simulink model "meam_simulink"  (R2020a)
settings: Solver=FixedStepAuto  StartTime=0.0  StopTime=10.0  FixedStep=0.0001  RelTol=1e-3
undefined symbols (not defined in the file): cnc_comp, ctc_switch, ctrl_at_end, ctrl_space, delta, ea_set_1, ea_set_2, ee_att_1, ee_att_2, f_des, force_ffwd, fp_1, fp_2, frc_comp, grv_comp, ip_1, ip_2, K, Kc, Kd, Kdf, Ki, Kif, Km, Kp, Kpf, orn_at_norm, prdc_frc, q_posIni, q_posIni_1, robot_model_1, robot_model_2, rpt_num_1, rpt_num_2, Sf_diag, spr_comp, switch_val, Sx_diag, tf_1, tf_2, trj_at_end, trj_profile_1, trj_profile_2, trj_space_1, trj_space_2, trj_type_1, trj_type_2
libraries: simulink x2, vrlib x1
(part 2 of 4)

== system meam_simulink/Subsystem/End-to-Base ==
  y : Inport  PortDimensions=6
  des : Inport  Port=2  PortDimensions=30
  fbk : Inport  Port=3  PortDimensions=30
  Constant2 : Constant  Value=ctrl_at_end
  Demux : Demux  Outputs=[12;18]
  Demux1 : Demux  Outputs=[12;18]
  Demux2 : Demux  Outputs=[12;6]
  Switch : Switch  Criteria=u2 > Threshold
  Terminator : Terminator
  Terminator1 : Terminator
  computed torque switch : Constant  Value=ctc_switch
  spatialTrnsE2B : MATLAB Function  TreatAsAtomicUnit=on
  u : Outport  PortDimensions=6
  wires:
  y/1 -> spatialTrnsE2B/5(u), Switch/3
  spatialTrnsE2B/1(y) -> Switch/1
  Constant2/1 -> Switch/2
  des/1 -> Demux/1
  Demux/1 -> spatialTrnsE2B/1(q)
  Demux/2 -> spatialTrnsE2B/2(x)
  Switch/1 -> u/1
  computed torque switch/1 -> spatialTrnsE2B/4(ctc_switch)
  fbk/1 -> Demux1/1
  Demux1/2 -> Demux2/1
  Demux2/2 -> spatialTrnsE2B/3(v)
  Demux1/1 -> Terminator/1
  Demux2/1 -> Terminator1/1

== system meam_simulink/Subsystem/End-to-Base Wrench ==
  y : Inport  PortDimensions=6
  des : Inport  Port=2  PortDimensions=30
  Constant2 : Constant  Value=ctrl_at_end
  Demux : Demux  Outputs=[12;18]
  Switch : Switch  Criteria=u2 > Threshold
  Terminator : Terminator
  spatialTrnsE2B : MATLAB Function  TreatAsAtomicUnit=on
  u : Outport  PortDimensions=6
  wires:
  y/1 -> Switch/3, spatialTrnsE2B/2(f_desE)
  spatialTrnsE2B/1(f_des) -> Switch/1
  Constant2/1 -> Switch/2
  des/1 -> Demux/1
  Demux/2 -> spatialTrnsE2B/1(x)
  Switch/1 -> u/1
  Demux/1 -> Terminator/1

== system meam_simulink/Subsystem/Error ==
  des : Inport  PortDimensions=30
  fbk : Inport  Port=2  PortDimensions=30
  Demux : Demux  Outputs=[12;18]
  Demux1 : Demux  Outputs=[12;18]
  MATLAB Function : MATLAB Function  TreatAsAtomicUnit=on
  Sum : Sum  Inputs=|+-
  Switch : Switch  Criteria=u2 > Threshold
  control_space : Constant  Value=ctrl_space
  e : Outport
  wires:
  fbk/1 -> Demux1/1
  des/1 -> Demux/1
  control_space/1 -> Switch/2
  MATLAB Function/1(y) -> Switch/1
  Demux/1 -> Sum/1
  Demux1/1 -> Sum/2
  Sum/1 -> Switch/3
  Demux/2 -> MATLAB Function/1(des)
  Demux1/2 -> MATLAB Function/2(fbk)
  Switch/1 -> e/1

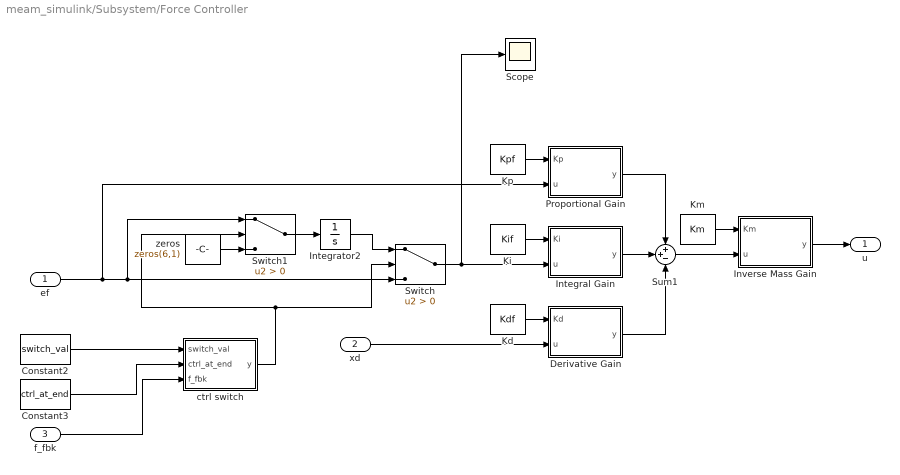
== system meam_simulink/Subsystem/Force Controller ==
  ef : Inport
  xd : Inport  Port=2
  f_fbk : Inport  Port=3
  Constant2 : Constant  Value=switch_val
  Constant3 : Constant  Value=ctrl_at_end
  Derivative Gain : MATLAB Function  TreatAsAtomicUnit=on
  Integral Gain : MATLAB Function  TreatAsAtomicUnit=on
  Integrator2 : Integrator
  Inverse Mass Gain : MATLAB Function  TreatAsAtomicUnit=on
  Kd : Constant  Value=Kdf
  Ki : Constant  Value=Kif
  Km : Constant  Value=Km
  Kp : Constant  Value=Kpf
  Proportional Gain : MATLAB Function  TreatAsAtomicUnit=on
  Scope : Scope
  Sum1 : Sum  Inputs=++-
  Switch : Switch  Criteria=u2 > Threshold
  Switch1 : Switch  Criteria=u2 > Threshold
  ctrl switch : MATLAB Function  TreatAsAtomicUnit=on
  zeros : Constant  Value=zeros(6,1)
  u : Outport
  wires:
  Proportional Gain/1(y) -> Sum1/1
  Integral Gain/1(y) -> Sum1/2
  ef/1 -> Switch/3, Switch1/1, Proportional Gain/2(u)
  Kp/1 -> Proportional Gain/1(Kp)
  Ki/1 -> Integral Gain/1(Ki)
  Kd/1 -> Derivative Gain/1(Kd)
  Derivative Gain/1(y) -> Sum1/3
  xd/1 -> Derivative Gain/2(u)
  Inverse Mass Gain/1(y) -> u/1
  Sum1/1 -> Inverse Mass Gain/2(u)
  Km/1 -> Inverse Mass Gain/1(Km)
  Constant3/1 -> ctrl switch/2(ctrl_at_end)
  Constant2/1 -> ctrl switch/1(switch_val)
  f_fbk/1 -> ctrl switch/3(f_fbk)
  Switch1/1 -> Integrator2/1
  Integrator2/1 -> Switch/1
  zeros/1 -> Switch1/3
  ctrl switch/1(y) -> Switch/2, Switch1/2
  Switch/1 -> Scope/1, Integral Gain/2(u)

== system meam_simulink/Subsystem/Kin Trns ==
  u : Inport
  q_fbk : Inport  Port=2
  Demux : Demux  Outputs=[6;6]
  Demux1 : Demux  Outputs=[12;18]
  MATLAB Function : MATLAB Function  TreatAsAtomicUnit=on
  Switch : Switch  Criteria=u2 > Threshold
  Terminator1 : Terminator
  computed torque switch : Constant  Value=ctc_switch
  control space : Constant  Value=ctrl_space
  end-effector attach : Constant  Value=ee_att_1
  robot_model : Constant  Value=robot_model_1
  y : Outport
  wires:
  u/1 -> Switch/3, MATLAB Function/4(u)
  robot_model/1 -> MATLAB Function/1(robot_model)
  Demux/1 -> MATLAB Function/5(q_pos)
  control space/1 -> Switch/2
  q_fbk/1 -> Demux1/1
  Demux1/1 -> Demux/1
  Demux/2 -> MATLAB Function/6(q_vel)
  Demux1/2 -> Terminator1/1
  Switch/1 -> y/1
  MATLAB Function/1(tau) -> Switch/1
  computed torque switch/1 -> MATLAB Function/3(ctc_switch)
  end-effector attach/1 -> MATLAB Function/2(ee_att)

== system meam_simulink/Subsystem/Motion Controller ==
  e : Inport
  Demux1 : Demux  Outputs=2
  Derivative Gain : MATLAB Function  TreatAsAtomicUnit=on
  Integral Gain : MATLAB Function  TreatAsAtomicUnit=on
  Integrator2 : Integrator
  Inverse Mass Gain : MATLAB Function  TreatAsAtomicUnit=on
  Kd : Constant  Value=Kd
  Ki : Constant  Value=Ki
  Km : Constant  Value=Km
  Kp : Constant  Value=Kp
  Proportional Gain : MATLAB Function  TreatAsAtomicUnit=on
  Scope : Scope
  Sum1 : Sum  Inputs=+++
  u : Outport
  wires:
  Derivative Gain/1(y) -> Sum1/3
  Proportional Gain/1(y) -> Sum1/1
  Integrator2/1 -> Integral Gain/2(u)
  Integral Gain/1(y) -> Sum1/2
  Demux1/2 -> Derivative Gain/2(u)
  e/1 -> Demux1/1
  Demux1/1 -> Scope/1, Proportional Gain/2(u), Integrator2/1
  Kp/1 -> Proportional Gain/1(Kp)
  Ki/1 -> Integral Gain/1(Ki)
  Kd/1 -> Derivative Gain/1(Kd)
  Km/1 -> Inverse Mass Gain/1(Km)
  Inverse Mass Gain/1(y) -> u/1
  Sum1/1 -> Inverse Mass Gain/2(u)

== system meam_simulink/Subsystem/Selective Sum ==
  um : Inport  PortDimensions=6
  uf : Inport  Port=2  PortDimensions=6
  f_fbk : Inport  Port=3  PortDimensions=6
  Constant : Constant  Value=Sx_diag
  Constant1 : Constant  Value=Sf_diag
  Constant2 : Constant  Value=switch_val
  Constant3 : Constant  Value=ctrl_at_end
  MATLAB Function : MATLAB Function  TreatAsAtomicUnit=on
  Out1 : Outport  PortDimensions=6
  wires:
  uf/1 -> MATLAB Function/6(uf)
  um/1 -> MATLAB Function/1(um)
  MATLAB Function/1(y) -> Out1/1
  Constant/1 -> MATLAB Function/2(Sx_diag)
  Constant1/1 -> MATLAB Function/5(Sf_diag)
  Constant2/1 -> MATLAB Function/3(switch_val)
  f_fbk/1 -> MATLAB Function/7(f_fbk)
  Constant3/1 -> MATLAB Function/4(ctrl_at_end)

== system meam_simulink/Subsystem1/Acc Switch ==
  In1 : Inport
  In2 : Inport  Port=2
  Demux : Demux  Outputs=2
  Sum : Sum  Inputs=++|
  Switch : Switch  Criteria=u2 > Threshold
  Switch1 : Switch  Criteria=u2 > Threshold
  computed torque switch : Constant  Value=ctc_switch
  control space : Constant  Value=ctrl_space
  Out1 : Outport
  wires:
  Sum/1 -> Switch/1
  computed torque switch/1 -> Switch/2
  Switch/1 -> Out1/1
  In1/1 -> Switch/3, Sum/1
  Switch1/1 -> Sum/2
  In2/1 -> Demux/1
  Demux/1 -> Switch1/3
  control space/1 -> Switch1/2
  Demux/2 -> Switch1/1

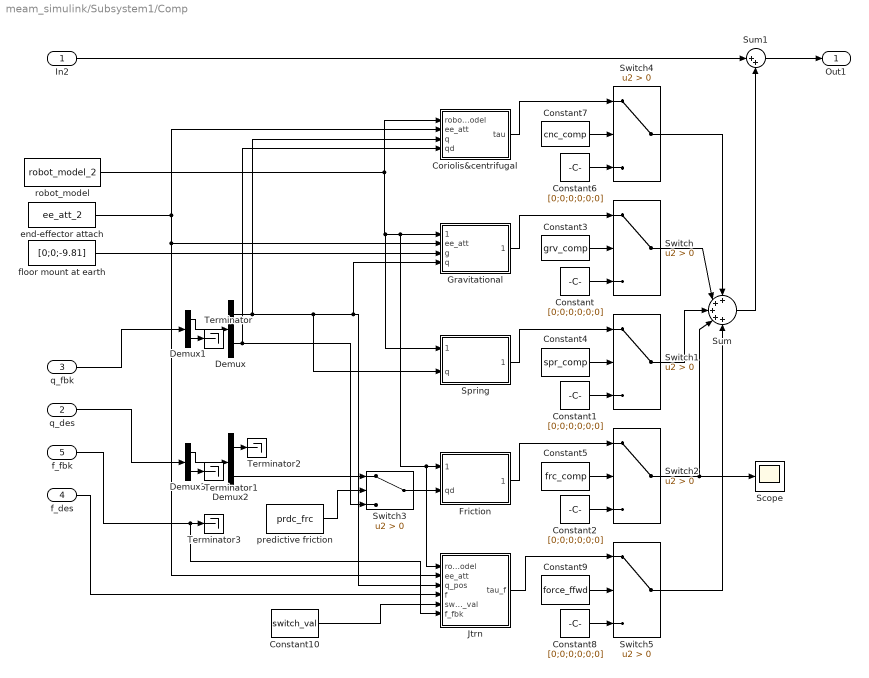
== system meam_simulink/Subsystem1/Comp ==
  In2 : Inport
  q_des : Inport  Port=2
  q_fbk : Inport  Port=3
  f_des : Inport  Port=4
  f_fbk : Inport  Port=5
  Constant{,1..2,6,8} (5 alike) : Constant  Value=[0;0;0;0;0;0]
  Constant10 : Constant  Value=switch_val
  Constant3 : Constant  Value=grv_comp
  Constant4 : Constant  Value=spr_comp
  Constant5 : Constant  Value=frc_comp
  Constant7 : Constant  Value=cnc_comp
  Constant9 : Constant  Value=force_ffwd
  Coriolis&centrifugal : MATLAB Function  TreatAsAtomicUnit=on
  Demux : Demux  Outputs=2
  Demux1 : Demux  Outputs=[12;18]
  Demux2 : Demux  Outputs=2
  Demux3 : Demux  Outputs=[12;18]
  Friction : MATLAB Function  TreatAsAtomicUnit=on
  Gravitational : MATLAB Function  TreatAsAtomicUnit=on
  Jtrn : MATLAB Function  TreatAsAtomicUnit=on
  Scope : Scope
  Spring : MATLAB Function  TreatAsAtomicUnit=on
  Sum : Sum  Inputs=+++++
  Sum1 : Sum  Inputs=|++
  Switch{,1..5} (6 alike) : Switch  Criteria=u2 > Threshold
  Terminator{,1..3} (4 alike) : Terminator
  end-effector attach : Constant  Value=ee_att_2
  floor mount at earth : Constant  Value=[0;0;-9.81]
  predictive friction : Constant  Value=prdc_frc
  robot_model : Constant  Value=robot_model_2
  Out1 : Outport
  wires:
  Sum/1 -> Sum1/2
  Sum1/1 -> Out1/1
  In2/1 -> Sum1/1
  Constant7/1 -> Switch4/2
  Switch1/1 -> Sum/3
  Coriolis&centrifugal/1(tau) -> Switch4/1
  Switch4/1 -> Sum/1
  Demux2/2 -> Switch3/1
  f_fbk/1 -> Jtrn/6(f_fbk), Terminator3/1
  Constant6/1 -> Switch4/3
  q_des/1 -> Demux3/1
  Demux2/1 -> Terminator2/1
  Constant/1 -> Switch/3
  Demux3/2 -> Terminator1/1
  Demux1/1 -> Demux/1
  Constant5/1 -> Switch2/2
  predictive friction/1 -> Switch3/2
  Constant4/1 -> Switch1/2
  Switch/1 -> Sum/2
  robot_model/1 -> Coriolis&centrifugal/1(robot_model), Jtrn/1(robot_model), Friction/1(robot_model), Gravitational/1(robot_model), Spring/1(robot_model)
  q_fbk/1 -> Demux1/1
  Demux3/1 -> Demux2/1
  Spring/1(tau_spr) -> Switch1/1
  Switch2/1 -> Scope/1, Sum/4
  Constant1/1 -> Switch1/3
  Demux/1 -> Jtrn/3(q_pos), Gravitational/4(q), Spring/2(q), Coriolis&centrifugal/3(q)
  Friction/1(tau_frc) -> Switch2/1
  Gravitational/1(tau_grv) -> Switch/1
  Demux1/2 -> Terminator/1
  Demux/2 -> Coriolis&centrifugal/4(qd), Switch3/3
  Constant3/1 -> Switch/2
  Constant2/1 -> Switch2/3
  Switch3/1 -> Friction/2(qd)
  Constant8/1 -> Switch5/3
  Constant9/1 -> Switch5/2
  Jtrn/1(tau_f) -> Switch5/1
  Switch5/1 -> Sum/5
  floor mount at earth/1 -> Gravitational/3(g)
  end-effector attach/1 -> Jtrn/2(ee_att), Gravitational/2(ee_att), Coriolis&centrifugal/2(ee_att)
  f_des/1 -> Jtrn/4(f)
  Constant10/1 -> Jtrn/5(switch_val)

== system meam_simulink/Subsystem1/Dyn Trns ==
  u : Inport
  q_fbk : Inport  Port=2
  Demux : Demux  Outputs=[6;6]
  Demux1 : Demux  Outputs=[12;18]
  MATLAB Function : MATLAB Function  TreatAsAtomicUnit=on
  Switch : Switch  Criteria=u2 > Threshold
  Terminator : Terminator
  Terminator1 : Terminator
  computed torque switch : Constant  Value=ctc_switch
  end-effector attach : Constant  Value=ee_att_2
  robot_model : Constant  Value=robot_model_2
  y : Outport
  wires:
  u/1 -> Switch/3, MATLAB Function/3(u)
  robot_model/1 -> MATLAB Function/1(robot_model)
  q_fbk/1 -> Demux1/1
  Demux/1 -> MATLAB Function/4(q)
  Demux1/1 -> Demux/1
  Demux1/2 -> Terminator1/1
  Demux/2 -> Terminator/1
  Switch/1 -> y/1
  computed torque switch/1 -> Switch/2
  MATLAB Function/1(tau) -> Switch/1
  end-effector attach/1 -> MATLAB Function/2(ee_att)

== system meam_simulink/Subsystem1/Error ==
  des : Inport
  fbk : Inport  Port=2
  Demux : Demux  Outputs=[12;18]
  Demux1 : Demux  Outputs=[12;18]
  MATLAB Function : MATLAB Function  TreatAsAtomicUnit=on
  Sum : Sum  Inputs=|+-
  Switch : Switch  Criteria=u2 > Threshold
  control_space : Constant  Value=ctrl_space
  e : Outport
  wires:
  fbk/1 -> Demux1/1
  des/1 -> Demux/1
  control_space/1 -> Switch/2
  MATLAB Function/1(y) -> Switch/1
  Demux/1 -> Sum/1
  Demux1/1 -> Sum/2
  Sum/1 -> Switch/3
  Demux/2 -> MATLAB Function/1(des)
  Demux1/2 -> MATLAB Function/2(fbk)
  Switch/1 -> e/1

== system meam_simulink/Subsystem1/Force Controller ==
  ef : Inport
  xd : Inport  Port=2
  D Controller : MATLAB Function  TreatAsAtomicUnit=on
  Demux : Demux  Outputs=[12;18]
  Demux1 : Demux  Outputs=[12;6]
  I Controller : MATLAB Function  TreatAsAtomicUnit=on
  Integrator2 : Integrator
  Kd : Constant  Value=Kdf
  Ki : Constant  Value=Kif
  Kp : Constant  Value=Kpf
  P Controller : MATLAB Function  TreatAsAtomicUnit=on
  Sum1 : Sum  Inputs=+++
  Terminator : Terminator
  Terminator1 : Terminator
  u : Outport
  wires:
  Sum1/1 -> u/1
  P Controller/1(y) -> Sum1/1
  Integrator2/1 -> I Controller/2(u)
  I Controller/1(y) -> Sum1/2
  ef/1 -> P Controller/2(u), Integrator2/1
  Kp/1 -> P Controller/1(Kp)
  Ki/1 -> I Controller/1(Ki)
  Kd/1 -> D Controller/1(Kd)
  Demux/2 -> Demux1/1
  Demux1/2 -> D Controller/2(u)
  Demux1/1 -> Terminator/1
  D Controller/1(y) -> Sum1/3
  xd/1 -> Demux/1
  Demux/1 -> Terminator1/1

== system meam_simulink/Subsystem1/Kin Trns ==
  u : Inport
  q_fbk : Inport  Port=2
  Demux : Demux  Outputs=[6;6]
  Demux1 : Demux  Outputs=[12;18]
  MATLAB Function : MATLAB Function  TreatAsAtomicUnit=on
  Switch : Switch  Criteria=u2 > Threshold
  Terminator1 : Terminator
  computed torque switch : Constant  Value=ctc_switch
  control space : Constant  Value=ctrl_space
  end-effector attach : Constant  Value=ee_att_2
  robot_model : Constant  Value=robot_model_2
  y : Outport
  wires:
  u/1 -> Switch/3, MATLAB Function/4(u)
  robot_model/1 -> MATLAB Function/1(robot_model)
  Demux/1 -> MATLAB Function/5(q_pos)
  control space/1 -> Switch/2
  q_fbk/1 -> Demux1/1
  Demux1/1 -> Demux/1
  Demux/2 -> MATLAB Function/6(q_vel)
  Demux1/2 -> Terminator1/1
  Switch/1 -> y/1
  MATLAB Function/1(tau) -> Switch/1
  computed torque switch/1 -> MATLAB Function/3(ctc_switch)
  end-effector attach/1 -> MATLAB Function/2(ee_att)

== system meam_simulink/Subsystem1/Motion Controller ==
  e : Inport
  D Controller : MATLAB Function  TreatAsAtomicUnit=on
  Demux1 : Demux  Outputs=2
  I Controller : MATLAB Function  TreatAsAtomicUnit=on
  Integrator2 : Integrator
  Kd : Constant  Value=Kd
  Ki : Constant  Value=Ki
  Kp : Constant  Value=Kp
  P Controller : MATLAB Function  TreatAsAtomicUnit=on
  Scope : Scope
  Sum1 : Sum  Inputs=+++
  u : Outport
  wires:
  Sum1/1 -> u/1
  D Controller/1(y) -> Sum1/3
  P Controller/1(y) -> Sum1/1
  Integrator2/1 -> I Controller/2(u)
  I Controller/1(y) -> Sum1/2
  Demux1/2 -> D Controller/2(u)
  e/1 -> Demux1/1
  Demux1/1 -> Scope/1, P Controller/2(u), Integrator2/1
  Kp/1 -> P Controller/1(Kp)
  Ki/1 -> I Controller/1(Ki)
  Kd/1 -> D Controller/1(Kd)

== system meam_simulink/Subsystem1/Selective Sum ==
  um : Inport  PortDimensions=6
  uf : Inport  Port=2  PortDimensions=6
  f_fbk : Inport  Port=3  PortDimensions=6
  Constant : Constant  Value=Sx_diag
  Constant1 : Constant  Value=Sf_diag
  Constant2 : Constant  Value=switch_val
  MATLAB Function : MATLAB Function  TreatAsAtomicUnit=on
  Out1 : Outport  PortDimensions=6
  wires:
  uf/1 -> MATLAB Function/5(uf)
  um/1 -> MATLAB Function/1(um)
  MATLAB Function/1(y) -> Out1/1
  Constant/1 -> MATLAB Function/2(Sx_diag)
  Constant1/1 -> MATLAB Function/4(Sf_diag)
  Constant2/1 -> MATLAB Function/3(switch_val)
  f_fbk/1 -> MATLAB Function/6(f_fbk)

== system meam_simulink/Trajectory Generation/Enabled Subsystem ==
  In1 : Inport
  Enable : EnablePort
  Out1 : Outport
  wires:
  In1/1 -> Out1/1

== system meam_simulink/Subsystem/Compliance/Subsystem ==
  In1 : Inport
  Demux : Demux  Outputs=6
  Mux : Mux  Inputs=6
  Transfer Fcn{,1..5} (6 alike) : TransferFcn  Denominator=[1e-4 1]
  Out1 : Outport
  wires:
  Transfer Fcn2/1 -> Mux/3
  In1/1 -> Demux/1
  Transfer Fcn/1 -> Mux/1
  Demux/2 -> Transfer Fcn1/1
  Demux/4 -> Transfer Fcn3/1
  Demux/1 -> Transfer Fcn/1
  Transfer Fcn5/1 -> Mux/6
  Transfer Fcn1/1 -> Mux/2
  Demux/6 -> Transfer Fcn5/1
  Transfer Fcn4/1 -> Mux/5
  Demux/5 -> Transfer Fcn4/1
  Transfer Fcn3/1 -> Mux/4
  Demux/3 -> Transfer Fcn2/1
  Mux/1 -> Out1/1

== matlab function meam_simulink/Trajectory Generation/MATLAB Function1 ==
  data: ip input; fp input; t input; tf input; trj_space input; ea_set input; trj_type input; trj_profile input; rpt_num input; q_pos output; robot_model input; ee_att input; trj_at_end input; q_vel output; q_acc output; x_pos output; x_vel output; ref input; x_acc output
function [q_pos,q_vel,q_acc,x_pos,x_vel,x_acc] = trj_gen(ip,fp,t,tf,trj_space,ea_set,trj_type,trj_profile,rpt_num,robot_model,ee_att,trj_at_end,ref)
    
    if t > tf
        t = tf;
    end

    if trj_space == 0
        
        [r_pos,r_vel,r_acc] = p2pTrj(t,tf,trj_profile);
        
        qi = ip;
        qf = fp;
        
        D = qf - qi;

        q_pos = qi + r_pos*D;
        q_vel = r_vel*D;
        q_acc = r_acc*D;
        
        % forward kinematics
        
        [a_i,alpha_i,d_i,thetaPlus_i] = kinematicParametersOrigin(robot_model);

        [T0_h,~] = forwardGeometry(a_i,alpha_i,d_i,thetaPlus_i+q_pos);

        d_e = getEElength(ee_att);

        Tn_E = [1 0 0 0
                0 1 0 0
                0 0 1 d_e
                0 0 0 1];
            
        T0_E = T0_h(:,:,end)*Tn_E;
    
        t_pos = T0_E(1:3,4);

        J_e = jacobian(a_i,d_i,d_e,q_pos);

        r_posDC = [T0_E(1:3,1);T0_E(1:3,2);T0_E(1:3,3)];

        J_eDot = jacobianDot(a_i,d_i,d_e,q_pos,q_vel);

        x_pos = [t_pos;r_posDC];
        x_vel = J_e*q_vel;
        x_acc = J_eDot*q_vel + J_e*q_acc;

    else
        
        if trj_at_end == 0
            p_ei = ip(1:3);
            r_ei = ip(4:6);
            R = eye(3);
            p = zeros(3,1);
            Sp = zeros(3,3);
        else
            p_ei = zeros(3,1);
            r_ei = zeros(3,1);
            
            p = ip(1:3);
            r_ea = ip(4:6);
            R = getRotMatfromEA(r_ea,ea_set);
            Sp = SkewSym(p);
            
%             X = [R Sp*R;0 R];
        end
        p_ef = fp(1:3);
        r_ef = fp(4:6);

        Dp = p_ef - p_ei;
        Dr = r_ef - r_ei;
        
        if trj_type ~= 1
            
            [r_pos,r_vel,r_acc] = p2pTrj(t,tf,trj_profile);
            
            t_pos   = p_ei + r_pos*Dp;
            r_posEA = r_ei + r_pos*Dr;

            t_vel   = r_vel*Dp;
            r_velEA = r_vel*Dr;

            t_acc   = r_acc*Dp;
            r_accEA = r_acc*Dr;

        else
            
            period = tf/rpt_num;
            
            Dp = p_ef - p_ei;
            Dr = r_ef - r_ei;
            
            f = (2*pi) / period;
            t_velMax = (Dp*f) / 2.0;
            r_velMax = (Dr*f) / 2.0;
            
            t_pos = p_ei + t_velMax * (1 - cos(f*t)) / f;
            t_vel = t_velMax * sin(f*t);
            t_acc = t_velMax * f * cos(f*t);
            
            r_posEA = r_ei + r_velMax * (1 - cos(f*t)) / f;
            r_velEA = r_velMax * sin(f*t);
            r_accEA = r_velMax * f * cos(f*t);
            
        end
        
        R_e     = getRotMatfromEA(r_posEA,ea_set);

        r_posDC = [R_e(:,1);R_e(:,2);R_e(:,3)];

        E_R     = getE_Rmatrix(r_posEA,ea_set);

        r_velAV = E_R*r_velEA;

        E_RDot  = getE_RDotmatrix(r_posEA,r_velEA,ea_set);
        
        r_accAV = E_RDot*r_velEA+E_R*r_accEA;
        
        if trj_at_end == 0  % Base Frame
            t_posDes = t_pos;
            t_velDes = t_vel;
            t_accDes = t_acc;
        else                % Tool Frame
            t_posDes = [    R(1,1)*t_pos(1)+R(1,2)*t_pos(2)+R(1,3)*t_pos(3)+p(1)
                            R(2,1)*t_pos(1)+R(2,2)*t_pos(2)+R(2,3)*t_pos(3)+p(2)
                            R(3,1)*t_pos(1)+R(3,2)*t_pos(3)+R(3,3)*t_pos(3)+p(3)    ];
            t_velDes = R*t_vel+Sp*R*r_velAV;
            t_accDes = R*t_acc+Sp*R*r_accAV;
        end
        
        x_pos = [t_posDes;r_posDC];        
        x_vel = [t_velDes;r_velAV];
        x_acc = [t_accDes;r_accAV];
        
        % inverse kinematics
        p_e = t_posDes;
        
        T0_E = [R_e, p_e;zeros(1,3) 1];

        q_ref = ref(1:6);
        
        [a_i,alpha_i,d_i,thetaPlus_i] = kinematicParametersOrigin(robot_model);

        d_e = getEElength(ee_att);

        q_pos = invGeo(T0_E,a_i,alpha_i,d_i,d_e,thetaPlus_i,q_ref,1);

        J_eInv = inv_jacobian(a_i,d_i,d_e,q_pos);

        q_vel = J_eInv*x_vel;
        
        J_eDot = jacobianDot(a_i,d_i,d_e,q_pos,q_vel);

        q_acc = J_eInv * (x_acc - (J_eDot*q_vel));
    end
    
    function [r_pos,r_vel,r_acc] = p2pTrj(t,tf,trj_profile)
        
        switch trj_profile
            case 1
                r_pos = t/tf;
                r_vel = 1/tf;
                r_acc = 0;
            case 2
                r_pos = 3*(t/tf)^2 - 2*(t/tf)^3;
                r_vel = 6*(t/tf^2) - 6*(t^2/tf^3);
                r_acc = 6/tf^2 - 12*(t/tf^3);
            case 3
                r_pos = 10*(t/tf)^3 - 15*(t/tf)^4 + 6*(t/tf)^5;
                r_vel = 30*(t^2/tf^3) - 60*(t^3/tf^4) + 30*(t^4/tf^5);
                r_acc = 60*(t/tf^3) - 180*(t^2/tf^4) + 120*(t^3/tf^5);
            case 4
                if t <= tf/2
                    r_pos = 2*(t/tf)^2;
                    r_vel = 4*(t/tf^2);
                    r_acc = 4/tf^2;
                else
                    r_pos = -1 + 4*(t/tf) - 2*(t/tf)^2;
                    r_vel = 4/tf - 4*(t/tf^2);
                    r_acc = -4/tf^2;
                end
            otherwise
                r_pos = 0;
                r_vel = 0;
                r_acc = 0;
        end
        
    end

    function E_R = getE_Rmatrix(r_posEA,eulerSet)
        
        phi = r_posEA(1,1);
        tht = r_posEA(2,1);

        % rotational mapping matrix E_R for euler angles
        E_R = zeros(3,3);
        switch eulerSet
            case 2 % ZYZ
                E_R(1,1) = 0.0;
                E_R(1,2) = -sin(phi);
                E_R(1,3) = cos(phi) * sin(tht);
                E_R(2,1) = 0.0;
                E_R(2,2) = cos(phi);
                E_R(2,3) = sin(phi) * sin(tht);
                E_R(3,1) = 1.0;
                E_R(3,2) = 0.0;
                E_R(3,3) = cos(tht);
            case 3 % ZYX
                E_R(1,1) = 0.0;
                E_R(1,2) = -sin(phi);
                E_R(1,3) = cos(tht) * cos(phi);
                E_R(2,1) = 0.0;
                E_R(2,2) = cos(phi);
                E_R(2,3) = cos(tht) * sin(phi);
                E_R(3,1) = 1.0;
                E_R(3,2) = 0.0;
                E_R(3,3) = -sin(tht);
            case 4 % XYZ
                E_R(1,1) = 1.0;
                E_R(1,2) = 0.0;
                E_R(1,3) = sin(tht);
                E_R(2,1) = 0.0;
                E_R(2,2) = cos(phi);
                E_R(2,3) = -cos(tht) * sin(phi);
                E_R(3,1) = 0.0;
                E_R(3,2) = sin(phi);
                E_R(3,3) = cos(phi) * cos(tht);
            otherwise % ZXZ
                E_R(1,1) = 0.0;
                E_R(1,2) = cos(phi);
                E_R(1,3) = sin(phi) * sin(tht);
                E_R(2,1) = 0.0;
                E_R(2,2) = sin(phi);
                E_R(2,3) = -cos(phi) * sin(tht);
                E_R(3,1) = 1.0;
                E_R(3,2) = 0.0;
                E_R(3,3) = cos(tht);
        end
    end

    function E_RDot = getE_RDotmatrix(r_posEA,r_velEA,eulerSet)
        
        phi = r_posEA(1);
        tht = r_posEA(2);

        phidot = r_velEA(1);
        thtdot = r_velEA(2);

        E_RDot = zeros(3,3);
        switch (eulerSet)
            case 2 % ZYZ
            	E_RDot(1,1) = 0.0;
            	E_RDot(1,2) = -phidot * cos(phi);
            	E_RDot(1,3) = thtdot * cos(phi)*cos(tht) - phidot * sin(phi)*sin(tht);
            	E_RDot(2,1) = 0.0;
            	E_RDot(2,2) = -phidot * sin(phi);
            	E_RDot(2,3) = thtdot * cos(tht)*sin(phi) + phidot * cos(phi)*sin(tht);
            	E_RDot(3,1) = 0.0;
            	E_RDot(3,2) = 0.0;
            	E_RDot(3,3) = -thtdot * sin(tht);
            case 3 % ZYX
            	E_RDot(1,1) = 0.0;
            	E_RDot(1,2) = -phidot * cos(phi);
            	E_RDot(1,3) = -phidot * cos(tht)*sin(phi) - thtdot * cos(phi)*sin(tht);
            	E_RDot(2,1) = 0.0;
            	E_RDot(2,2) = -phidot * sin(phi);
            	E_RDot(2,3) = phidot * cos(phi)*cos(tht) - thtdot * sin(phi)*sin(tht);
            	E_RDot(3,1) = 0.0;
            	E_RDot(3,2) = 0.0;
            	E_RDot(3,3) = -thtdot * cos(tht);
            case 4 %XYZ:
            	E_RDot(1,1) = 0.0;
            	E_RDot(1,2) = 0.0;
            	E_RDot(1,3) = thtdot * cos(tht);
            	E_RDot(2,1) = 0.0;
            	E_RDot(2,2) = -phidot * sin(phi);
            	E_RDot(2,3) = -phidot * cos(phi)*cos(tht) + thtdot * sin(phi)*sin(tht);
            	E_RDot(3,1) = 0.0;
            	E_RDot(3,2) = phidot * cos(phi);
            	E_RDot(3,3) = -phidot * cos(tht)*sin(phi) - thtdot * cos(phi)*sin(tht);
            otherwise % ZXZ
            	E_RDot(1,1) = 0.0;
            	E_RDot(1,2) = -phidot * sin(phi);
            	E_RDot(1,3) = thtdot * cos(tht)*sin(phi) + phidot * cos(phi)*sin(tht);
            	E_RDot(2,1) = 0.0;
            	E_RDot(2,2) = phidot * cos(phi);
            	E_RDot(2,3) = -thtdot * cos(phi)*cos(tht) + phidot * sin(phi)*sin(tht);
            	E_RDot(3,1) = 0.0;
            	E_RDot(3,2) = 0.0;
            	E_RDot(3,3) = -thtdot * sin(tht);
        end
    end

%     function R_dot = getR0_6dotMatrix(q_pos,q_vel)
%         
%         C1 = cos(q_pos(1));
%         C4 = cos(q_pos(4));
%         C5 = cos(q_pos(5));
%         C6 = cos(q_pos(6));
% 
%         S1 = sin(q_pos(1));
%         S4 = sin(q_pos(4));
%         S5 = sin(q_pos(5));
%         S6 = sin(q_pos(6));
% 
%         C2p3 = cos(q_pos(2) + q_pos(3));
%         S2p3 = sin(q_pos(2) + q_pos(3));
% 
%         qd1 = q_vel(1);
%         qd2 = q_vel(2);
%         qd3 = q_vel(3);
%         qd4 = q_vel(4);
%         qd5 = q_vel(5);
%         qd6 = q_vel(6);
% 
%         R_dot = zeros(3,3);
%         
%         R_dot(1,1) = -(C1 * (C5*C6*S4 + C4*S6) * qd1) + S1 * (C6*S2p3*S5 + C2p3 * (-(C4*C5*C6) + S4*S6)) * qd1 ...
%                     - S1 * ((C4*C5*C6 - S4*S6) * qd4 - C6*S4*S5 * qd5 + (C4*C6 - C5*S4*S6) * qd6) + C1 * (-(C2p3*C6*S5 * (qd2 + qd3)) ...
%                     - S2p3 * (C4*C5*C6 - S4*S6) * (qd2 + qd3) - C5*C6*S2p3 * qd5 + S2p3*S5*S6 * qd6 - C2p3 * ((C5*C6*S4 + C4*S6) * qd4 ...
%                     + C4*C6*S5 * qd5 + (C6*S4 + C4*C5*S6) * qd6));
% 	    R_dot(1,2) = -(C6 * ((C1*C4 - C2p3*S1*S4) * qd1 - C1*S2p3*S4 * (qd2 + qd3) + (C1*C2p3*C4 - S1*S4) * qd4)) ...
%                     + S6 * (C1*C5*S4 * qd1 + S1 * (C2p3*C4*C5 - S2p3*S5) * qd1 + C4*C5*S1 * qd4 - S1*S4*S5 * qd5 ...
%                     + C1 * (C4*C5*S2p3 * (qd2 + qd3) + C2p3*S5 * (qd2 + qd3) + C2p3*C5*S4 * qd4 + C5*S2p3 * qd5 ...
%                     + C2p3*C4*S5 * qd5)) + C6 * (C5*S1*S4 + C1 * (-(C2p3*C4*C5) + S2p3*S5)) * qd6 + (C4*S1 + C1*C2p3*S4) * S6 * qd6;
% 	    R_dot(1,3) = -(C1*S4*S5 * qd1) - S1 * (C5*S2p3 + C2p3*C4*S5) * qd1 - C4*S1*S5 * qd4 - C5*S1*S4 * qd5 ...
%                     + C1 * (C2p3*C5 * (qd2 + qd3) - C4*S2p3*S5 * (qd2 + qd3) - C2p3*S4*S5 * qd4 + C2p3*C4*C5 * qd5 - S2p3*S5 * qd5);
% 	    R_dot(2,1) = -(C1*C6*S2p3*S5 * qd1) - S1 * (C5*C6*S4 + C4*S6) * qd1 + C1*C2p3 * (C4*C5*C6 - S4*S6) * qd1 ...
%                     - C2p3*C6*S1*S5 * (qd2 + qd3) - S1*S2p3 * (C4*C5*C6 - S4*S6) * (qd2 + qd3) - C5*C6*S1*S2p3 * qd5 + S1*S2p3*S5*S6 * qd6 ...
%                     - C2p3*S1 * ((C5*C6*S4 + C4*S6) * qd4 + C4*C6*S5 * qd5 + (C6*S4 + C4*C5*S6) * qd6) + C1 * ((C4*C5*C6 - S4*S6) * qd4 ...
%                     - C6*S4*S5 * qd5 + (C4*C6 - C5*S4*S6) * qd6);
% 	    R_dot(2,2) = C1*S2p3*S5*S6 * qd1 - C1*C2p3 * (C6*S4 + C4*C5*S6) * qd1 + S1 * (-(C4*C6) + C5*S4*S6) * qd1 ...
%                     + C2p3*S1*S5*S6 * (qd2 + qd3) + S1*S2p3 * (C6*S4 + C4*C5*S6) * (qd2 + qd3) + C5*S1*S2p3*S6 * qd5 ...
%                     + C6*S1*S2p3*S5 * qd6 - C1 * ((C6*S4 + C4*C5*S6) * qd4 - S4*S5*S6 * qd5 + (C5*C6*S4 + C4*S6) * qd6) ...
%                     - C2p3*S1 * ((C4*C6 - C5*S4*S6) * qd4 - C4*S5*S6 * qd5 + (C4*C5*C6 - S4*S6) * qd6);
% 	    R_dot(2,3) = C1*C5*S2p3 * qd1 + C2p3*C5*S1 * (qd2 + qd3) + S5 * ((C1*C2p3*C4 - S1*S4) * qd1 ...
%                     - C4*S1*S2p3 * (qd2 + qd3) + (C1*C4 - C2p3*S1*S4) * qd4) + C5 * (C2p3*C4*S1 + C1*S4) * qd5 - S1*S2p3*S5 * qd5;
% 	    R_dot(3,1) = C2p3*S4*S6 * (qd2 + qd3) + C4*S2p3*S6 * qd4 - C6 * (C2p3*C4*C5 * (qd2 + qd3) - S2p3*S5 * (qd2 + qd3) ...
%                     - C5*S2p3*S4 * qd4 + C2p3*C5 * qd5 - C4*S2p3*S5 * qd5) + C6*S2p3*S4 * qd6 + (C4*C5*S2p3 + C2p3*S5) * S6 * qd6;
% 	    R_dot(3,2) = C2p3*C6*S4 * (qd2 + qd3) + C4*C6*S2p3 * qd4 + S6 * (C2p3*C4*C5 * (qd2 + qd3) - S2p3*S5 * (qd2 + qd3) ...
%                     - C5*S2p3*S4 * qd4 + C2p3*C5 * qd5 - C4*S2p3*S5 * qd5) + C6 * (C4*C5*S2p3 + C2p3*S5) * qd6 - S2p3*S4*S6 * qd6;
% 	    R_dot(3,3) = -(C5*S2p3 * (qd2 + qd3)) - C2p3*C4*S5 * (qd2 + qd3) + S2p3*S4*S5 * qd4 - C4*C5*S2p3 * qd5 ...
%                     - C2p3*S5 * qd5;
%                 
%     end

    function S = SkewSym(r)
        S = [   0   , -r(3) ,  r(2)
                r(3),  0   	, -r(1)
               -r(2),  r(1)	,  0  	];
    end

end

== matlab function meam_simulink/Subsystem/Comp/Coriolis&centrifugal ==
  data: robot_model input; ee_att input; q input; qd input; tau output
function tau = b_hat(robot_model,ee_att,q,qd)

    tau = zeros(6,1);
    
    [a_i,alpha_i,d_i,thetaPlus_i] = kinematicParametersOrigin(robot_model);

    d_e = getEElength(ee_att);

    [~,Th_i] = forwardGeometry(a_i,alpha_i,d_i,thetaPlus_i+q);

    Tn_E = [1 0 0 0
            0 1 0 0
            0 0 1 d_e
            0 0 0 1];

    Th_i(:,:,end) = Th_i(:,:,end)*Tn_E;
    
    Rh_i = zeros(3,3,6+1);
    Rh_i(:,:,1:6) = Th_i(1:3,1:3,:);

    [m_i,ri_i_ci,Ii_i] = staticInertialParameters(robot_model,ee_att);

    rh_h_i = zeros(3,1,6+1); % +1 because of prcNE
    ci_i = zeros(3,1,6);
    for j = 1:6
        % origin i-1 to i on frame i-1
        rh_h_i(:,:,j) = Th_i(1:3,4,j);
        ci_i(:,:,j) = m_i(j) * ri_i_ci(:,:,j);
    end
    
    q_obj.Rh_i = Rh_i;
    p_obj.rh_h_i = rh_h_i;
    p_obj.m_i = m_i;
    p_obj.ci_i = ci_i;
    p_obj.Ii_i = Ii_i;

    tau = prcNE(p_obj,q_obj,qd,zeros(6,1),zeros(3,1));
    
end

== matlab function meam_simulink/Subsystem/Error/MATLAB Function ==
  data: y output; des input; fbk input
function y = getTaskSpcError(des,fbk)

    t_posDes = des(1:3);
    t_posFbk = fbk(1:3);
    
    x_velDes = des(13:18);
    x_velFbk = fbk(13:18);
    
    e_trn = t_posDes-t_posFbk;

    r_des = [des(4:6) des(7:9) des(10:12)];
    r_fbk = [fbk(4:6) fbk(7:9) fbk(10:12)];

    e_rot = 0.5*(cross(r_fbk(:,1),r_des(:,1))+cross(r_fbk(:,2),r_des(:,2))+cross(r_fbk(:,3),r_des(:,3)));

    e_pos = [e_trn;e_rot];

    e_vel = x_velDes-x_velFbk;

    y = [e_pos;e_vel];
        
end

== matlab function meam_simulink/Subsystem/Selective Sum/MATLAB Function ==
  data: um input; y output; Sx_diag input; switch_val input; ctrl_at_end input; Sf_diag input; uf input; f_fbk input
function y = fcn(um,Sx_diag,switch_val,ctrl_at_end,Sf_diag,uf,f_fbk)
    
    y = zeros(6,1);
    Sx_i = Sx_diag;
    Sf_i = Sf_diag;

    if ctrl_at_end == 1
        fc_axis = 3;
    else
        fc_axis = 2;
    end
    
    if f_fbk(fc_axis) < switch_val
        Sx_i(fc_axis) = 1;
        Sf_i(fc_axis) = 0;
    end
    
%     if f_fbk(1) < switch_val
%         Sx_diag(1) = 1;
%         Sf_diag(1) = 0;
%     end
%     
%     Sx_i = Sx_diag;
%     Sf_i = Sf_diag;

    for i = 1:6
        y(i) = Sx_i(i)*um(i)+Sf_i(i)*uf(i);
    end

end

== matlab function meam_simulink/Subsystem/Kin Trns/MATLAB Function ==
  data: robot_model input; ee_att input; ctc_switch input; u input; tau output; q_pos input; q_vel input
function tau = kinematicTrans(robot_model,ee_att,ctc_switch,u,q_pos,q_vel)

    [a_i,~,d_i,~] = kinematicParametersOrigin(robot_model);

	d_e = getEElength(ee_att);

    if ctc_switch == 0
        J_e = jacobian(a_i,d_i,d_e,q_pos);

        tau = J_e'*u;
    else
        J_eDot = jacobianDot(a_i,d_i,d_e,q_pos,q_vel);
        J_eInv = inv_jacobian(a_i,d_i,d_e,q_pos);
        
        tau = J_eInv*(u-J_eDot*q_vel);
    end

end

== matlab function meam_simulink/Robot (Stäubli RX160)/fwd kin ==
  data: robot_model input; ee_att input; u input; y output
function y = fwdKin(robot_model,ee_att,u)

    q_pos = u(1:6);
    q_vel = u(7:12);
    
    [a_i,alpha_i,d_i,thetaPlus_i] = kinematicParametersOrigin(robot_model);
    
    d_e = getEElength(ee_att);

    [T0_h,~] = forwardGeometry(a_i,alpha_i,d_i,thetaPlus_i+q_pos);
    
    Tn_E = [1 0 0 0
            0 1 0 0
            0 0 1 d_e
            0 0 0 1];

    T0_E = T0_h(:,:,end)*Tn_E;

    t_pos = T0_E(1:3,4);

    J_e = jacobian(a_i,d_i,d_e,q_pos);
    
    r_posDC = [T0_E(1:3,1);T0_E(1:3,2);T0_E(1:3,3)];
    
    x_pos = [t_pos;r_posDC];
    x_vel = J_e*q_vel;
    
    y = [x_pos;x_vel];

%     function x = spring_model_func(f)
% 
%         p1 =   2.015e-13;
%         p2 =   7.036e-11;
%         p3 =   9.407e-09;
%         p4 =    5.66e-07;
%         p5 =   1.201e-05;
%         p6 =    0.000136;
%         p7 =  -1.792e-07;
% 
%         if f >= 0
%             x = 0;
%         elseif f >= -109.743
%             x = p1*f^6+p2*f^5+p3*f^4+p4*f^3+p5*f^2+p6*f+p7;
%         else
%             x = -0.0219;
%         end
% 
%     end
end

== matlab function meam_simulink/Environment/MATLAB Function ==
  data: K input; delta input; u input size=18; t input; f output; x output
function [f,x] = fcn(K,delta,u,t)

    obs_x = 0.8+delta*sin(2*t);
    x_pos = u(1:3);
    
    f = zeros(6,1);
    x = zeros(3,1);
    
    if (x_pos(1) > obs_x)
        f = +[K*(x_pos(1)-obs_x);0;0;0;0;0];
%         f = +[K;0;0;0;0;0];
    end
    
%     % floor
%     if (x_pos(3) < 0)
%         f = [0;0;K*x_pos(3);0;0;0];
%     end
    
    x = [obs_x+0.01;1.25;0.6];

end

== matlab function meam_simulink/Subsystem/Force Controller/Integral Gain ==
  data: Ki input; u input size=6; y output size=6
function y = fcn(Ki,u)

    f = zeros(6,1);
    
    f(1) = Ki(1)*u(1);
    f(2) = Ki(2)*u(2);
    f(3) = Ki(3)*u(3);
    f(4) = Ki(4)*u(4);
    f(5) = Ki(5)*u(5);
    f(6) = Ki(6)*u(6);

y = f;

== matlab function meam_simulink/Subsystem/Force Controller/Proportional Gain ==
  data: Kp input; u input size=6; y output size=6
function y = fcn(Kp,u)

    f = zeros(6,1);
    
    f(1) = Kp(1)*u(1);
    f(2) = Kp(2)*u(2);
    f(3) = Kp(3)*u(3);
    f(4) = Kp(4)*u(4);
    f(5) = Kp(5)*u(5);
    f(6) = Kp(6)*u(6);

y = f;

== matlab function meam_simulink/Robot (Stäubli RX160)/Jtrn ==
  data: robot_model input; ee_att input; q_pos input size=6; tau_f output size=6; f input
function tau_f = forceTorque(robot_model,ee_att,q_pos,f)

    [a_i,~,d_i,~] = kinematicParametersOrigin(robot_model);

    d_e = getEElength(ee_att);

    J_e = jacobian(a_i,d_i,d_e,q_pos);

    tau_f = J_e'*f;

% tau_f = zeros(6,1);
        
end

== matlab function meam_simulink/Measurement/fwd kin ==
  data: robot_model input; ee_att input; u input; y output
function y = fwdKin(robot_model,ee_att,u)

    q_pos = u(1:6);
    q_vel = u(7:12);
    
    x_pos = zeros(12,1);
    x_vel = zeros(6,1);
    
    [a_i,alpha_i,d_i,thetaPlus_i] = kinematicParametersOrigin(robot_model);
    
    d_e = getEElength(ee_att);

    [T0_h,~] = forwardGeometry(a_i,alpha_i,d_i,thetaPlus_i+q_pos);
    
    Tn_E = [1 0 0 0
            0 1 0 0
            0 0 1 d_e
            0 0 0 1];

    T0_E = T0_h(:,:,end)*Tn_E;

    t_pos = T0_E(1:3,4);

    J_e = jacobian(a_i,d_i,d_e,q_pos);
    
    r_posDC = [T0_E(1:3,1);T0_E(1:3,2);T0_E(1:3,3)];
    
    x_pos = [t_pos;r_posDC];
    x_vel = J_e*q_vel;
    
    y = [x_pos;x_vel];

end

== matlab function meam_simulink/Subsystem/Comp/Jtrn ==
  data: robot_model input; ee_att input; q_pos input size=6; tau_f output size=6; f input; switch_val input; f_fbk input
function tau_f = forceTorque(robot_model,ee_att,q_pos,f,switch_val,f_fbk)

    fc_axis = 2; % task frame 1: x, 2: y, 3: z
    
    if f_fbk(fc_axis) < switch_val
        f = zeros(6,1);
    end
    
    [a_i,~,d_i,~] = kinematicParametersOrigin(robot_model);

    d_e = getEElength(ee_att);

    J_e = jacobian(a_i,d_i,d_e,q_pos);

    tau_f = J_e'*f;

% tau_f = zeros(6,1);
        
end

== matlab function meam_simulink/Robot (Stäubli RX160)/Spring ==
  data: robot_model input; q input size=6; tau_spr output size=6
function tau_spr = spring(robot_model,q)

    % Integrated spring and friction models from feedback
    tau_spr = springModel(robot_model,q);
    
    function tau = springModel(robot_model,q)

        r = 0.08;
        L = 0.728;

        if robot_model == 2
            Pc  = 5314;
            a0  = deg2rad(-0.8458);
            k   = 23950;
        elseif robot_model == 3
            Pc  = 4897;
            a0  = deg2rad(-1.186);
            k   = 19690;
        else
            Pc  = 0;
            a0  = 0;
            k   = 0;
        end

        x0 = sqrt(r^2+(r+L)^2-2*r*(r+L)*cos(a0+q(2)))-L;

        B1E = r*sin(a0+q(2));
        A2G = ((L+r)*B1E)./(L+x0);

        % F = k*x+Pc;

        F1 = k*x0;
        F2 = Pc*ones(1,length(x0));

        tau1 = F1.*A2G;
        tau2 = F2.*A2G;

        tau = zeros(6,1);
        tau(2) = tau1 + tau2;

    end

end

== matlab function meam_simulink/Animation/fwd kin ==
  data: u input; r1 output; r2 output; r3 output; r4 output; r5 output; r6 output
function [r1,r2,r3,r4,r5,r6] = fcn(u)

%     [a_i,~,d_i,~] = kinematicParametersOrigin(robot_model);

    r1 = [0;1; 0;u(1)];
    r2 = [0;0;-1;u(2)];
    r3 = [0;0;-1;u(3)];
    r4 = [0;1; 0;u(4)];
    r5 = [0;0;-1;u(5)];
    r6 = [0;1; 0;u(6)];

%     t1 = [0         d_i(1)  0]';
%     t2 = [a_i(2)    0       0]';
%     t3 = [0         a_i(3)	0]';
%     t4 = [0         0       0]';
%     t5 = [0         d_i(4)  0]';
%     t6 = [0         d_i(6)  0]';

end

== matlab function meam_simulink/Subsystem/Force Controller/Derivative Gain ==
  data: Kd input; u input size=6; y output size=6
function y = fcn(Kd,u)

    f = zeros(6,1);
    
    f(1) = Kd(1)*u(1);
    f(2) = Kd(2)*u(2);
    f(3) = Kd(3)*u(3);
    f(4) = Kd(4)*u(4);
    f(5) = Kd(5)*u(5);
    f(6) = Kd(6)*u(6);

y = f;

== matlab function meam_simulink/Robot (Stäubli RX160)/x_e ==
  data: ee_att_1 input; f_vec input; y output
function y = end_point(ee_att_1,f_vec)

    f = -f_vec(2);
    
    if ee_att_1 == 3
        if f > 0
            y = [0;0;0];
        elseif f < -109.8066
            y = [0;0;0.0219];
        else            
            y = [0;0;f/5014];
        end
    else
        y = [0;0;0];
    end    
    
end

== matlab function meam_simulink/Robot (Stäubli RX160)/Friction ==
  data: robot_model input; tau_frc output size=6; qd input size=6
function tau_frc = friction(robot_model,qd)

%     tau_frc = frictionViscousModel(robot_model,qd);
%     tau_frc = frictionVisCoulModel(robot_model,qd);
    tau_frc = frictionPWModel(robot_model,qd);
    
    function tau_frc = frictionPWModel(robot_model,qd)

        tau_frc = zeros(6,1);
        
        v = zeros(7,1);
        c = zeros(7,1);
        o = zeros(7,1);
        n = zeros(7,1);
        p = zeros(7,1);
        
        tau = zeros(7,1);
        vel = zeros(7,1);
        vel(1:6) = qd;
        vel(7) = qd(5)+qd(6);        

        if robot_model == 1 || robot_model == 2 || robot_model == 3
            v = [111.2  ;87.28  ;36.49  ;9.596  ;15.42  ;0.1652 ;6.564];    % Viscous
            c = [35.98  ;55.28  ;27.51  ;7.647  ;4.747  ;0.5175 ;2.805];    % Coulumb
            o = [0.9811 ;-4.794 ;-7.222 ;0.01566;0.7782 ;0.007565;-0.2884]; % Offset
%             n = [70109  ;120235 ;69500  ;15272  ;7953   ;1020   ;6193];     % Negative slop
%             p = [74033  ;101059 ;40612  ;15335  ;11066  ;1050   ;5040];     % Positive slop
%             n = [35110	;60161	;34768	;7641	;3984	;510	;3100];     % Negative slop
%             p = [37072  ;50573  ;20324  ;7672   ;5541   ;525    ;2523];     % Positive slop
%             n = [3611   ;6095   ;3510   ;773    ;412    ;51.2   ;316];     % Negative slop
%             p = [3807   ;5136   ;2065   ;776    ;568    ;52.7   ;258];     % Positive slop
            n = [461.2  ;688.0  ;383.8  ;85.91  ;55.11  ;5.265  ;37.50];     % Negative slop
            p = [480.8  ;592.1  ;239.4  ;86.22  ;70.67  ;5.416  ;31.73];     % Positive slop
        end
        
        for i = 1:7
            if (vel(i) > -1e-1 && vel(i) <= 0)
                tau(i) = n(i)*vel(i);
            elseif  (vel(i) > 0 && vel(i) <= 1e-1)
                tau(i) = p(i)*vel(i);
            else
                tau(i) = v(i)*vel(i)+c(i)*sign(vel(i))+o(i);
            end
        end
        
        tau_frc(1) = tau(1);
        tau_frc(2) = tau(2);
        tau_frc(3) = tau(3);
        tau_frc(4) = tau(4);
        tau_frc(5) = tau(5) + tau(7);
        tau_frc(6) = tau(6) + tau(7);

    end

%     function tau_frc = frictionViscousModel(robot_model,qd)
%     
%         tau_frc = zeros(6,1);
%         
%         if robot_model == 2 || robot_model == 3
%             tau_frc(1) = 133.7*qd(1);
%             tau_frc(2) = 121.8*qd(2);
%             tau_frc(3) = 53.69*qd(3);
%             tau_frc(4) = 14.38*qd(4);
% %             tau_frc(5) = 18.39*qd(5);
% %             tau_frc(6) = 14.71*qd(6);
%             
%             % Coupling
%             tau_frc_a = 18.39*qd(5);
%             tau_frc_b = 0.4887*qd(6);
%             tau_frc_c = 7.44*(qd(5)+qd(6));
% 
%             tau_frc(5) = tau_frc_a + tau_frc_c;
%             tau_frc(6) = tau_frc_b + tau_frc_c;
%     
%         end
%         
%     end

%     function tau_frc = frictionVisCoulModel(robot_model,qd)
% 
%         tau_frc = zeros(6,1);
% 
%         if robot_model == 2
%             tau_frc(1) = 111.2*qd(1) + 35.98*sign(qd(1)) + 0.9811;
%             tau_frc(2) = 87.28*qd(2) + 55.28*sign(qd(2)) - 4.794;
%             tau_frc(3) = 36.49*qd(3) + 27.51*sign(qd(3)) - 7.222;
%             tau_frc(4) = 9.596*qd(4) + 7.647*sign(qd(4)) + 0.01566;
% 
%             % Coupling
%             tau_frc_a = 15.42*qd(5) + 4.747*sign(qd(5)) + 0.7782;
%             tau_frc_b = 0.1652*qd(6) + 0.5175*sign(qd(6)) + 0.007565;
%             tau_frc_c = 6.564*(qd(5)+qd(6)) + 2.805*sign(qd(5)+qd(6)) - 0.2884;
% 
%             tau_frc(5) = tau_frc_a + tau_frc_c;
%             tau_frc(6) = tau_frc_b + tau_frc_c;
%         end
% 
%     end

    % function tau_frc = frictionModel(qd)
    % 
    % 	tau_a_bl_P = [ 35, 70, 15, 6.36, 5.015867, 0.20, 0.187356 ];
    % 	tau_a_bl_N = [ -36.95, -85.95, -36.0, -6.41, -4.1, 1.18, -2.1 ];
    % 
    % 	q_dot_striebeck_P = [ 0.26, 0.078, 0.09, 0.06, 0.06, 1.10, 0.05 ];
    % 	q_dot_striebeck_N = [ 0.26, 0.3, 0.9, 0.72, 0.072, 4.0, 0.2 ];
    % 
    % 	delta_a_P = [ 0.8, 0.28, 0.35, 0.57, 0.57, 0.80, 0.30 ];
    % 	delta_a_N = [ 0.4, 0.21, 0.465, 0.5, 0.34, 1.30, 0.34 ];
    % 
    % 	c_v_P = [ 150, 132, 68, 20.737, 24.529614, 17.758244 ];
    % 	c_v_N = [ -140.0, -118.5, -58.0, -17.5, -22.0, -18.860045 ];
    % 
    % 	delta_v_P = [ 0.24, 0.352, 0.48, 0.56, 0.411378, 0.300846 ];
    % 	delta_v_N = [ 0.24, 0.28, 0.30, 0.46, 0.30, 0.315 ];
    % 
    % 	tau_v_l_P = -0.9;
    % 	tau_v_l_N = -2; %//0.08;
    % 
    % 	q_dot_l_P = 5.0;
    % 	q_dot_l_N = -8.0;
    % 
    %     tau_frc = zeros(6,1);
    %     for j = 1:4
    %         if (qd(j) > 0)
    %             tau_frc(j) = tau_a_bl_P(j)*exp(-power((qd(j)/q_dot_striebeck_P(j)), delta_a_P(j))) ...
    %                     + c_v_P(j)*power(qd(j), (1 - delta_v_P(j)));
    %         elseif (qd(j) < 0)
    %             tau_frc(j) = tau_a_bl_N(j)*exp(-power(abs(qd(j)/q_dot_striebeck_N(j)), delta_a_N(j))) ...
    %                     + c_v_N(j)*power(abs(qd(j)), (1 - delta_v_N(j)));
    %         else
    %             tau_frc(j) = 0;
    %         end
    %     end
    % 
    %     if (qd(4) > 0)
    %         tau_a = tau_a_bl_P(4)*exp(-power((qd(4)/q_dot_striebeck_P(4)), delta_a_P(4))) ...
    %                 + c_v_P(4)*power(qd(4), (1 - delta_v_P(4)));
    %     elseif (qd(4) < 0)
    %         tau_a = tau_a_bl_N(4)*exp(-power((abs(qd(4))/q_dot_striebeck_N(4)), delta_a_N(4))) ...
    %                 + c_v_N(4)*power(abs(qd(4)), (1 - delta_v_N(4)));
    %     else
    %         tau_a = 0;
    %     end
    % 
    %     if (qd(5) > 0)
    %         tau_b = tau_a_bl_P(5)*exp(-power((qd(5)/q_dot_striebeck_P(5)), delta_a_P(5))) ...
    %                 + tau_v_l_P*(1 - exp(-(qd(5)/q_dot_l_P)));
    %     elseif (qd(5) < 0)
    %         tau_b = tau_a_bl_N(5)*exp(-power((abs(qd(5))/q_dot_striebeck_N(5)), delta_a_N(5))) ...
    %                 + tau_v_l_N*(1 - exp(-abs(qd(5))/q_dot_l_N));
    %     else
    %         tau_b = 0;
    %     end
    % 
    %     qd7 = qd(4) + qd(5);
    %     if (qd7 > 0)
    %         tau_c = tau_a_bl_P(6)*exp(-power((qd7/q_dot_striebeck_P(6)), delta_a_P(6))) ...
    %                 + c_v_P(5)*power(qd7, (1 - delta_v_P(5)));
    %     elseif (qd7 < 0)
    %         tau_c = tau_a_bl_N(6)*exp(-power((abs(qd7)/q_dot_striebeck_N(6)), delta_a_N(6))) ...
    %                 + c_v_N(5)*power(abs(qd7), (1 - delta_v_N(5)));
    %     else
    %         tau_c = 0;
    %     end
    % 
    %     tau_frc(4) = tau_a + tau_c;
    %     tau_frc(5) = tau_b + tau_c;
    %     
    % end

end

== matlab function meam_simulink/Environment/MATLAB Function2 ==
  data: x1 input; ee_att_1 input; x2 input size=18; K input; f output
function f = fcn(x1,ee_att_1,x2,K)

    origin2 = [-0.28;2.43;0];
    obs_y = origin2(2)+x2(2);
    x_pos = x1(1:3);
    
    f = zeros(6,1);
    
    obj_xP = 0.32;
    obj_xN = 0.32;
    obj_yP = 0.32;
    obj_yN = 0.32;
    
    col_x = x_pos(1) < (origin2(1)+x2(1)+obj_xP) && x_pos(1) > (origin2(1)+x2(1)-obj_xN);
    col_y = x_pos(2) > obs_y;
    col_z = x_pos(3) < (origin2(3)+x2(3)+obj_yP) && x_pos(3) > (origin2(3)+x2(3)-obj_yN);
    
    d = x_pos(2)-obs_y;
    
    if ee_att_1 == 3
        if d < 0.0219
            K = 5014;
        end
    end
    
    if (col_x && col_y && col_z)
        f = [0;K*d;0;0;0;0];
    end
    
%     % floor
%     if (x_pos(3) < 0)
%         f = [0;0;K*x_pos(3);0;0;0];
%     end
    
%     x = [obs_x+0.01;1.25;0.6];

end

== matlab function meam_simulink/Subsystem1/Comp/Coriolis&centrifugal ==
  data: robot_model input; ee_att input; q input; qd input; tau output
function tau = b_hat(robot_model,ee_att,q,qd)

    tau = zeros(6,1);
    
    [a_i,alpha_i,d_i,thetaPlus_i] = kinematicParametersOrigin(robot_model);

    d_e = getEElength(ee_att);

    [~,Th_i] = forwardGeometry(a_i,alpha_i,d_i,thetaPlus_i+q);

    Tn_E = [1 0 0 0
            0 1 0 0
            0 0 1 d_e
            0 0 0 1];

    Th_i(:,:,end) = Th_i(:,:,end)*Tn_E;
    
    Rh_i = zeros(3,3,6+1);
    Rh_i(:,:,1:6) = Th_i(1:3,1:3,:);

    [m_i,ri_i_ci,Ii_i] = staticInertialParameters(robot_model,ee_att);

    rh_h_i = zeros(3,1,6+1); % +1 because of prcNE
    ci_i = zeros(3,1,6);
    for j = 1:6
        % origin i-1 to i on frame i-1
        rh_h_i(:,:,j) = Th_i(1:3,4,j);
        ci_i(:,:,j) = m_i(j) * ri_i_ci(:,:,j);
    end
    
    q_obj.Rh_i = Rh_i;
    p_obj.rh_h_i = rh_h_i;
    p_obj.m_i = m_i;
    p_obj.ci_i = ci_i;
    p_obj.Ii_i = Ii_i;

    tau = prcNE(p_obj,q_obj,qd,zeros(6,1),zeros(3,1));
    
end
